simulink model "PTC_MBDS_DifferenceQuotient_Sample"  (R2013a)
settings: Solver=FixedStepDiscrete  StartTime=0.0  StopTime=100  FixedStep=Auto  RelTol=1e-3
undefined symbols (not defined in the file): sigbuilder_block
libraries: simulink_extras x1, PTC_MBDS_LIB x1
settings Model: Creator=uidl7367  LastModifiedBy=sundeep.tuteja
settings DataIOCC: SignalLoggingSaveFormat=ModelDataLogs
settings OptimizationCC: ExpressionDepthLimit=2147483647  InitFltsAndDblsToZero=on
settings DebuggingCC: SaveWithParameterizedLinksMsg=none  SignalResolutionControl=TryResolveAllWithWarning  SolverPrmCheckMsg=none  InheritedTsInSrcMsg=none  MultiTaskDSMMsg=warning  MultiTaskCondExecSysMsg=none  FcnCallInpInsideContextMsg=UseLocalSettings  StrictBusMsg=Warning
settings RTWCC: IncludeERTFirstTime=on
settings GRTTargetCC: TargetFcnLib=ansi_tfl_tmw.mat  CombineOutputUpdateFcns=off  GRTInterface=on

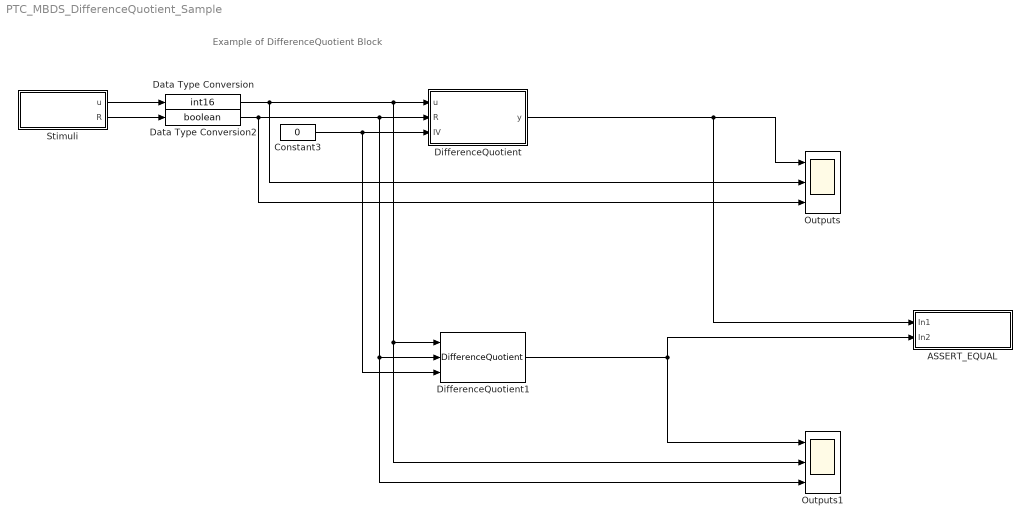
== system PTC_MBDS_DifferenceQuotient_Sample ==
  note: Example of DifferenceQuotient Block
  ASSERT_EQUAL : Subsystem
  Constant3 : Constant  InitFcn=|  Value=0  VectorParams1D=off  OutDataTypeStr=Inherit: Inherit via back propagation
      | if(exist('MBDS_BlockCallback', 'file'))
      |    MBDS_BlockCallback('Update', gcb);  
      | end
  Data Type Conversion : DataTypeConversion  InitFcn=|  OutDataTypeStr=int16  SaturateOnIntegerOverflow=on
      | try
      |    MBDS_BlockCallback('Update', gcb);
      | end
  Data Type Conversion2 : DataTypeConversion  InitFcn=|  OutDataTypeStr=boolean  SaturateOnIntegerOverflow=on
      | try
      |    MBDS_BlockCallback('Update', gcb);
      | end
  DifferenceQuotient : Subsystem  InitFcn=|  mask(DifferenceQuotient){MBDS_LibraryBlock=on, dT_Enabled=off, dT=1, R_Enabled=on, IV_Enabled=on, IV=0, MBDS_BlockVersion=05.40}
      | if(exist('MBDS_BlockCallback', 'file'))
      |    MBDS_BlockCallback('Update', gcb);
      | end
      mask prompts: MBDS_LibraryBlock "MBDS library block"; dT_Enabled "Show dT port"; dT "Sample rate (dT):"; R_Enabled "Show R port"; IV_Enabled "Show IV port"; IV "Initial value (IV):"; MBDS_BlockVersion "Block version:"
      mask help: Calculates the rate of change of the input signal over time.
      mask init:
      | if(exist('MBDS_BlockCallback', 'file'))
      |    MBDS_BlockCallback('Init', gcb);
      | else
      |    % Disable all mask parameters
      |    MaskEnables = get_param(gcb, 'MaskEnables');
      |    for k = [1:length(MaskEnables)]
      |       MaskEnables{k} = 'off';
      |    end
      |    if(~isequal(MaskEnables, get_param(gcb, 'MaskEnables')))
      |       set_param(gcb, 'MaskEnables', MaskEnables);
      |    end
      | end
      settings: AttributesFormatString=dT = %<dT>
      mask Help: eval(['open([workdir(''library_dir:''),''\Blockset\help\'',get_param(gcb,''MaskType''),''.html''])'])
      mask Callback dT_Enabled:
      | % Update mask parameter dialog
      | if(exist('MBDS_BlockCallback', 'file'))
      |    MBDS_BlockCallback('dT_Enabled', gcb);
      | end
      mask Callback dT:
      | % Adopt Value
      | if(exist('MBDS_BlockCallback', 'file'))
      |    MBDS_BlockCallback('dT', gcb);
      | end
      mask Callback R_Enabled:
      | % Update mask parameter dialog
      | if(exist('MBDS_BlockCallback', 'file'))
      |    MBDS_BlockCallback('R_Enabled', gcb);
      | end
      mask Callback IV_Enabled:
      | % Update mask parameter dialog
      | if(exist('MBDS_BlockCallback', 'file'))
      |    MBDS_BlockCallback('IV_Enabled', gcb);
      | end
      mask Callback IV:
      | % Adopt Value
      | if(exist('MBDS_BlockCallback', 'file'))
      |    MBDS_BlockCallback('IV', gcb);
      | end
      mask Display:
      | % Show icon or block text
      | if(exist('DifferenceQuotient.tif', 'file'))
      |    image(imread('DifferenceQuotient.tif','tif'), [0.295739348370927 0.17 0.378947368421053 0.66]);
      |    disp('')
      | else
      |    disp(sprintf('Difference\nQuotient'));
      | end
      | 
      | % Display port labels
      | port_label('input', 1, 'u');
      | port_label('input', 2, 'R');
      | port_label('input', 3, 'IV');
      | port_label('output', 1, 'y');
  DifferenceQuotient1 : PTC_MBDS_LIB/MBDS Standard Library/Extended Operations/Memory Blocks/DifferenceQuotient  dT_Enabled=off  dT=1  R_Enabled=on  IV_Enabled=on  IV=0  PTC_MBDS_BlockVersion=5.32  PTC_BlockType=PTC_MBDS_DifferenceQuotient
      settings: AttributesFormatString=dT = %<dT>
  Outputs : Scope  NumInputPorts=3
      settings: TimeRange=100  YMin=-2~-10~0  YMax=8~10~1  SampleInput=on  SampleTime=1
  Outputs1 : Scope  NumInputPorts=3
      settings: TimeRange=100  YMin=-2~-10~0  YMax=8~10~1  SampleInput=on  SampleTime=1
  Stimuli : Subsystem  Tag=STV Subsys  LoadFcn=sigbuilder_block('load');  StartFcn=sigbuilder_block('start');  StopFcn=sigbuilder_block('stop');  ClipboardFcn=sigbuilder_block('clipboard');  mask(Sigbuilder block){}
      mask help: Sigbuilder GUI
      mask init:
      | if ~strcmp(get_param(bdroot(gcb),'SimulationStatus'),'stopped') tuvar = sigbuilder_block('maskInit'); end
      settings: CopyFcn=sigbuilder_block('copy');  DeleteFcn=sigbuilder_block('delete');  ModelCloseFcn=sigbuilder_block('modelClose');  PreSaveFcn=sigbuilder_block('preSave');  PauseFcn=sigbuilder_block('pause')  ContinueFcn=sigbuilder_block('continue')  NameChangeFcn=sigbuilder_block('namechange');  OpenFcn=sigbuilder_block('open',[45 129.75 730.5 246 ]);  CloseFcn=sigbuilder_block('close');
      mask Display: plot(0,0,100,100,[10,10,40,40,10],[80,20,20,80,80],[40,10],[50,50], [40,27,10],[65,72,56],[40,25,25,10],[28,28,43,43]);
  wires:
  Stimuli/2(R) -> Data Type Conversion2/1
  Stimuli/1(u) -> Data Type Conversion/1
  Data Type Conversion/1 -> DifferenceQuotient1/1, Outputs1/2, DifferenceQuotient/1(u), Outputs/2
  DifferenceQuotient/1(y) -> ASSERT_EQUAL/1(In1), Outputs/1
  Data Type Conversion2/1 -> DifferenceQuotient1/2, Outputs1/3, DifferenceQuotient/2(R), Outputs/3
  Constant3/1 -> DifferenceQuotient1/3, DifferenceQuotient/3(IV)
  DifferenceQuotient1/1 -> ASSERT_EQUAL/2(In2), Outputs1/1

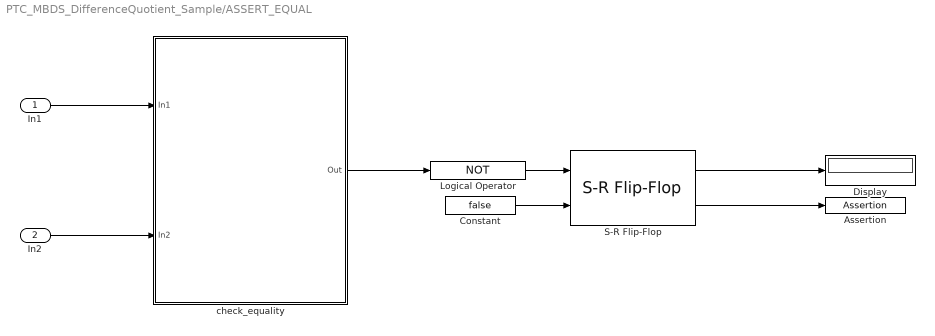
== system PTC_MBDS_DifferenceQuotient_Sample/ASSERT_EQUAL ==
  In1 : Inport
  In2 : Inport  Port=2
  Assertion : Assertion
  Constant : Constant  Value=false
  Display : Display
  Logical Operator : Logic  Operator=NOT  AllPortsSameDT=off  OutDataTypeStr=boolean
  S-R Flip-Flop : simulink_extras/Flip Flops/S-R Flip-Flop  initial_condition=0
  check_equality : MATLAB Function  TreatAsAtomicUnit=on
  wires:
  S-R Flip-Flop/1 -> Display/1
  check_equality/1(Out) -> Logical Operator/1
  Constant/1 -> S-R Flip-Flop/2
  S-R Flip-Flop/2 -> Assertion/1
  In2/1 -> check_equality/2(In2)
  In1/1 -> check_equality/1(In1)
  Logical Operator/1 -> S-R Flip-Flop/1

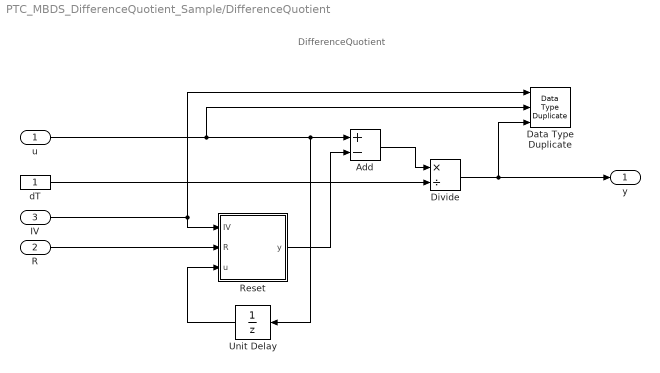
== system PTC_MBDS_DifferenceQuotient_Sample/DifferenceQuotient ==
  note: DifferenceQuotient
  u : Inport
  R : Inport  Port=2  OutDataTypeStr=boolean
  IV : Inport  Port=3
  Add : Sum  Inputs=+-  OutDataTypeStr=Inherit: Inherit via back propagation  SaturateOnIntegerOverflow=on
  Data Type Duplicate : DataTypeDuplicate  NumInputPorts=3
  Divide : Product  Inputs=*/  OutDataTypeStr=Inherit: Inherit via back propagation  SaturateOnIntegerOverflow=on
  Reset : Subsystem
  Unit Delay : UnitDelay  SampleTime=-1
  dT : Constant  OutDataTypeStr=Inherit: Inherit via back propagation
  y : Outport
  wires:
  Add/1 -> Divide/1
  Unit Delay/1 -> Reset/3(u)
  dT/1 -> Divide/2
  IV/1 -> Reset/1(IV), Data Type Duplicate/1
  Divide/1 -> y/1, Data Type Duplicate/3
  Reset/1(y) -> Add/2
  u/1 -> Data Type Duplicate/2, Unit Delay/1, Add/1
  R/1 -> Reset/2(R)

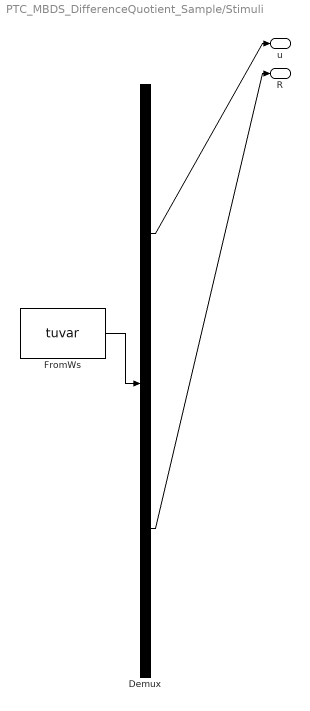
== system PTC_MBDS_DifferenceQuotient_Sample/Stimuli ==
  Demux : Demux  Tag=STV Demux  Outputs=2
  FromWs : FromWorkspace  Tag=STV FromWs  VariableName=tuvar  SampleTime=1  OutputAfterFinalValue=Holding final value
      SigBuilderData=|
      | common.afterFinalStr = 'Hold final value'
      | common.sampleTime = 1
      | dataSet.timeRange = [0 100]
      | dataSet.name = 'test data'
      | sbobj.Groups.Name = 'test data'
      | sbobj.Groups.Signals(1).Name = 'u'
      | sbobj.Groups.Signals(1).XData = [0 5 10 15 20 25 30 35 40 45 50 55 60 65 70 75 80 85 90 95 100]
      | sbobj.Groups.Signals(1).YData = [0 5.87770260526 9.51045063028 9.51073693746 5.87845217341 0.000926535896605 -5.87695298665 -9.51016424147 -9.51102316299 -5.87920169109 -0.00185307178526 5.87620331759 9.50987777101 9.51130930686 5.8799511583 0.002779607658 -5.87545359809 -9.50959121891 -9.51159536909 -5.88070057504 -0.00370614350688]
      | sbobj.Groups.Signals(2).Name = 'R'
      | sbobj.Groups.Signals(2).XData = [0 66.2 66.2 70.5 70.5 100]
      | sbobj.Groups.Signals(2).YData = [0 0 1 1 0 0]
  u : Outport  Tag=STV Outport
  R : Outport  Tag=STV Outport  Port=2
  wires:
  Demux/2 -> R/1
  Demux/1 -> u/1
  FromWs/1 -> Demux/1

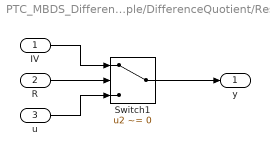
== system PTC_MBDS_DifferenceQuotient_Sample/DifferenceQuotient/Reset ==
  IV : Inport
  R : Inport  Port=2
  u : Inport  Port=3
  Switch1 : Switch  Criteria=u2 ~= 0  OutDataTypeStr=Inherit: Inherit via back propagation  InputSameDT=on
  y : Outport
  wires:
  u/1 -> Switch1/3
  Switch1/1 -> y/1
  IV/1 -> Switch1/1
  R/1 -> Switch1/2

== matlab function PTC_MBDS_DifferenceQuotient_Sample/ASSERT_EQUAL/check_equality ==
  data: In1 input; Out output; In2 input
function Out = check_equality(In1, In2)
%#codegen

Out = isequaln(In1, In2);

end
